simulink model "record_errp"  (R2015a)
settings: Solver=VariableStepDiscrete  StartTime=0.0  StopTime=inf  FixedStep=1/256  RelTol=1e-3
StartFcn:
  | coder.extrinsic('now');
  | coder.extrinsic('datestr');
  | coder.extrinsic('datetime');
  | coder.extrinsic('str2num');
  | 
  | nw = datetime('now');
  | 
  | year = str2double(datestr(nw,'yyyy'));
  | month = str2double(datestr(nw,'MM'));
  | day = str2double(datestr(nw,'dd'));
  | 
  | hr = str2double(datestr(nw,'HH'));
  | mn = str2double(datestr(nw,'MM'));
  | sec = str2double(datestr(nw,'SS'));
  | ms = str2double(datestr(nw,'FFF'));
  | 
  | time = [hr, mn, sec, ms];
  | disp(time)
undefined symbols (not defined in the file): currentCFG_record_errp_UR, UR
libraries: gUSBamplib x4, gtecHighspeedLib x2, dspnetwork x1
settings Model: ModifiedByFormat=g.tec  Creator=g.tec medical engineering  LastModifiedBy=g.tec
settings DataIOCC: LimitDataPoints=off  SignalLoggingSaveFormat=ModelDataLogs  SaveOutput=off  SignalLogging=off  SaveTime=off
settings OptimizationCC: ExpressionDepthLimit=2147483647  InitFltsAndDblsToZero=on
settings DebuggingCC: SaveWithParameterizedLinksMsg=none  UnderspecifiedInitializationDetection=Classic  MergeDetectMultiDrivingBlocksExec=none  SignalResolutionControl=TryResolveAllWithWarning  SolverPrmCheckMsg=warning  MultiTaskDSMMsg=warning  MultiTaskCondExecSysMsg=none  FcnCallInpInsideContextMsg=UseLocalSettings  UnconnectedInputMsg=none  UnconnectedOutputMsg=none  FrameProcessingCompatibilityMsg=none  StateNameClashWarn=warning
settings HardwareCC: ProdIntDivRoundTo=Floor  ProdEndianess=LittleEndian  ProdHWDeviceType=32-bit xPC Target (Intel Pentium)
settings RTWCC: SystemTargetFile=rtwin.tlc  TemplateMakefile=rtwintmf  Description=Real-Time Windows Target
settings TargetCC: TargetFcnLib=ansi_tfl_tmw.mat  ModelReferenceCompliant=off  CompOptLevelCompliant=off  MatFileLogging=on

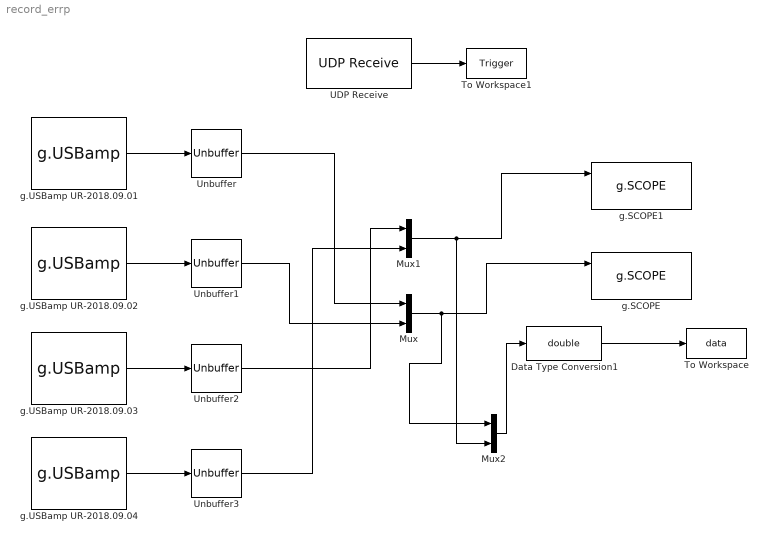
== system record_errp ==
  Data Type Conversion1 : DataTypeConversion  OutDataTypeStr=double
  Mux : Mux  Inputs=2
  Mux1 : Mux  Inputs=2
  Mux2 : Mux  Inputs=2
  To Workspace : ToWorkspace  VariableName=data  SampleTime=-1
  To Workspace1 : ToWorkspace  VariableName=Trigger  SaveFormat=Structure With Time  SampleTime=-1
  UDP Receive : dspnetwork/UDP Receive  localURL='0.0.0.0'  localPort=1234  remoteURL='127.0.0.1'  remotePort=-1  recvBufferSize=1024  dims=255  signalDatatype=uint8  isVarSize=on  showBlockingTime=off  blockingTime=0  sampletime=-1
  Unbuffer{,1..3} (4 alike) : Unbuffer
  g.SCOPE : gtecHighspeedLib/g.SCOPE
  g.SCOPE1 : gtecHighspeedLib/g.SCOPE
  g.USBamp UR-2018.09.01 : gUSBamplib/g.USBamp  Priority=2  cfg=currentCFG_record_errp_UR-2018.09.01.cfg  snr=UR-2018.09.01
  g.USBamp UR-2018.09.02 : gUSBamplib/g.USBamp  Priority=1  cfg=currentCFG_record_errp_UR-2018.09.02.cfg  snr=UR-2018.09.02
  g.USBamp UR-2018.09.03 : gUSBamplib/g.USBamp  Priority=1  cfg=currentCFG_record_errp_UR-2018.09.03.cfg  snr=UR-2018.09.03
  g.USBamp UR-2018.09.04 : gUSBamplib/g.USBamp  Priority=1  cfg=currentCFG_record_errp_UR-2018.09.04.cfg  snr=UR-2018.09.04
  wires:
  Data Type Conversion1/1 -> To Workspace/1
  g.USBamp UR-2018.09.01/1 -> Unbuffer/1
  g.USBamp UR-2018.09.02/1 -> Unbuffer1/1
  Unbuffer1/1 -> Mux/2
  Mux/1 -> Mux2/1, g.SCOPE/1
  Unbuffer/1 -> Mux/1
  g.USBamp UR-2018.09.03/1 -> Unbuffer2/1
  g.USBamp UR-2018.09.04/1 -> Unbuffer3/1
  UDP Receive/1 -> To Workspace1/1
  Unbuffer2/1 -> Mux1/1
  Unbuffer3/1 -> Mux1/2
  Mux1/1 -> Mux2/2, g.SCOPE1/1
  Mux2/1 -> Data Type Conversion1/1
